simulink model "Greg_Trans"  (Simulink 8.8)
settings: Solver=VariableStepAuto  StartTime=0.0  StopTime=10  RelTol=1e-3
values from neighbouring files (symbols this model uses):
  b = 0    [design_project_parameters.m]
  g = 9.81    [design_project_parameters.m]
  I = .0053    (= 0.0053)    [design_project_parameters.m]
  L = .235    (= 0.235)    [design_project_parameters.m]
  m = .1    (= 0.1)    [design_project_parameters.m]
  M = .9    (= 0.9)    [design_project_parameters.m]
settings Model: SuppressorTable=22 serialization::archive 11 0 3 0 0 0 0 0  Creator=greg  LastModifiedBy=greg
settings DataIOCC: LimitDataPoints=off  SaveFormat=Dataset  SignalLoggingSaveFormat=Dataset
settings OptimizationCC: LifeSpan=auto
settings DebuggingCC: UnderspecifiedInitializationDetection=Simplified  MergeDetectMultiDrivingBlocksExec=error  FcnCallInpInsideContextMsg=error  StateNameClashWarn=none  SFUnexpectedBacktrackingDiag=error  SFNoUnconditionalDefaultTransitionDiag=error  SFExecutionAtInitializationDiag=warning
settings HardwareCC: ProdBitPerPointer=64  ProdBitPerSizeT=64  ProdBitPerPtrDiffT=64  ProdLargestAtomicFloat=Float  ProdIntDivRoundTo=Zero  ProdEndianess=LittleEndian  ProdWordSize=64  ProdHWDeviceType=Intel->x86-64 (Windows64)
settings ModelReferenceCC: PropagateSignalLabelsOutOfModel=on
settings GRTTargetCC: TargetLangStandard=C99 (ISO)  GeneratePreprocessorConditionals=Use local settings  CombineOutputUpdateFcns=on  GRTInterface=off
settings ConfigComp: CovMetricSettings=dwe  CovHtmlReporting=off  CovSaveCumulativeToWorkspaceVar=off  CovSaveSingleToWorkspaceVar=off  CovExternalEMLEnable=on

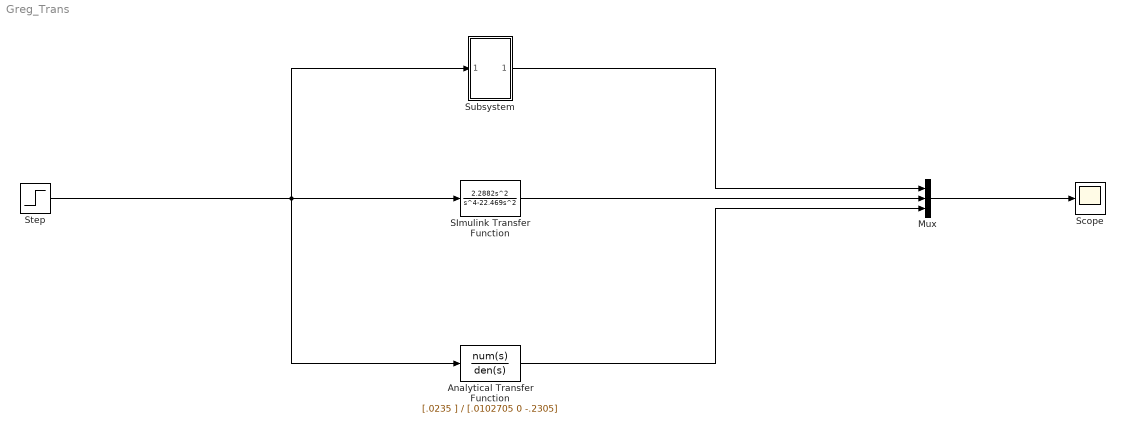
== system Greg_Trans ==
  "Analytical Transfer Function " : TransferFcn  Numerator=[.0235 ]  Denominator=[.0102705 0 -.2305]  ContinuousStateAttributes='Analytical'
  Mux : Mux  Inputs=3
  "SImulink Transfer Function " : TransferFcn  Numerator=[0 0 2.2882 0 0]  Denominator=[1 0 -22.469 0 0]
  Scope : Scope
  Step : Step  Time=0  SampleTime=0
  Subsystem : Subsystem
  wires:
  Step/1 -> "Analytical Transfer Function "/1, Subsystem/1(Force), "SImulink Transfer Function "/1
  Subsystem/1(Angle) -> Mux/1
  "SImulink Transfer Function "/1 -> Mux/2
  "Analytical Transfer Function "/1 -> Mux/3
  Mux/1 -> Scope/1

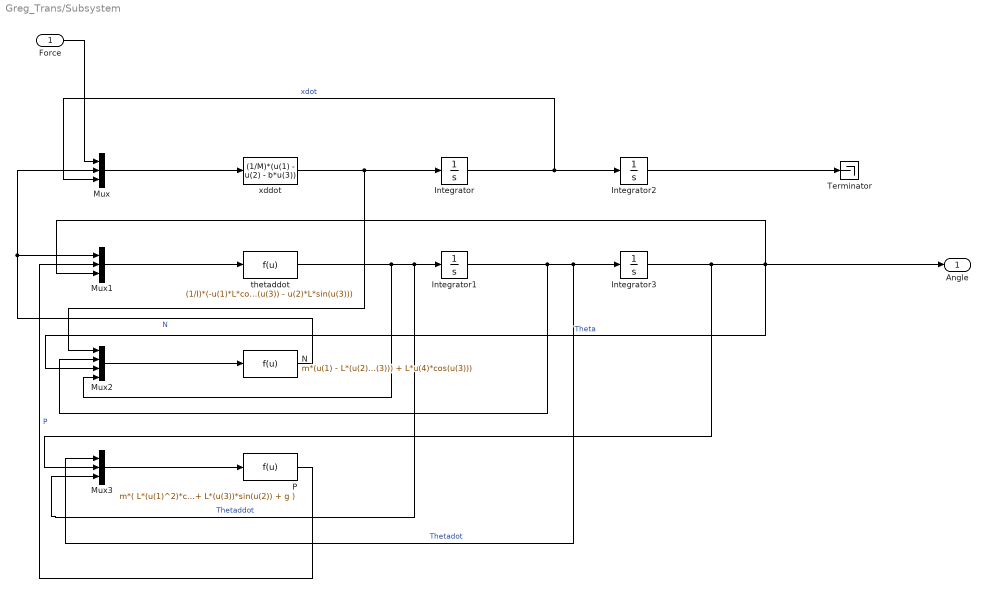
== system Greg_Trans/Subsystem ==
  Force : Inport
  Integrator : Integrator  ContinuousStateAttributes='xdot'
  Integrator1 : Integrator  ContinuousStateAttributes='thetadot'
  Integrator2 : Integrator  ContinuousStateAttributes='x'
  Integrator3 : Integrator  InitialCondition=pi  ContinuousStateAttributes='theta'
  Mux : Mux  Inputs=3
  Mux1 : Mux  Inputs=3
  Mux2 : Mux
  Mux3 : Mux  Inputs=3
  N : Fcn  Expr=m*(u(1) - L*(u(2)^2)*(sin(u(3))) + L*u(4)*cos(u(3)))
  P : Fcn  Expr=m*( L*(u(1)^2)*cos(u(2)) + L*(u(3))*sin(u(2)) + g )
  Terminator : Terminator
  thetaddot : Fcn  Expr=(1/I)*(-u(1)*L*cos(u(3)) - u(2)*L*sin(u(3)))
  "xddot " : Fcn  Expr=(1/M)*(u(1) - u(2) - b*u(3))
  Angle : Outport
  wires:
  Mux/1 -> "xddot "/1
  Integrator2/1 -> Terminator/1
  Integrator/1 -> Mux/3, Integrator2/1  "xdot"
  Mux1/1 -> thetaddot/1
  Mux2/1 -> N/1
  Mux3/1 -> P/1
  Force/1 -> Mux/1
  N/1 -> Mux/2, Mux1/1  "N"
  P/1 -> Mux1/2  "P"
  "xddot "/1 -> Mux2/1, Integrator/1
  Integrator3/1 -> Mux3/2, Angle/1, Mux2/3, Mux1/3  "Theta"
  Integrator1/1 -> Mux2/2, Mux3/1, Integrator3/1  "Thetadot"
  thetaddot/1 -> Mux2/4, Mux3/3, Integrator1/1  "Thetaddot"
